simulink model "px4demo_gps"  (R2017b)
settings: Solver=ode3  StartTime=0.0  StopTime=inf  RelTol=1e-3  EnableMultiTasking=on
PostLoadFcn:
  | Ts = 1/250;
undefined symbols (not defined in the file): RGBLED_COLOR_ENUM, RGBLED_MODE_ENUM
libraries: pixhawk_slib_sensors_actuators x2
Description:
  | PX4 PSP Demo Model - GPS
  | 
  | Example model to show how to use the GPS Input Block
settings Model: Creator=skuznick  LastModifiedBy=skuznick
settings SolverCC: PositivePriorityOrder=on
settings DataIOCC: LimitDataPoints=on  SaveFormat=Array
settings OptimizationCC: DefaultParameterBehavior=Inlined  LifeSpan=1  MaxStackSize=64
settings DebuggingCC: SolverPrmCheckMsg=warning  AllowSymbolicDim=off  SFUnexpectedBacktrackingDiag=warning  SFNoUnconditionalDefaultTransitionDiag=warning  SFExecutionAtInitializationDiag=none
settings HardwareCC: ProdBitPerPointer=32  ProdBitPerSizeT=32  ProdBitPerPtrDiffT=32  ProdLargestAtomicInteger=Long  ProdLargestAtomicFloat=Double  ProdWordSize=32  ProdHWDeviceType=ARM Compatible->ARM Cortex
settings ModelReferenceCC: PropagateSignalLabelsOutOfModel=off
settings SFSimCC: MATLABDynamicMemAlloc=off
settings RTWCC: SystemTargetFile=ert.tlc  TemplateMakefile=ert_default_tmf  GenerateReport=on  Toolchain=Pixhawk Toolchain  BuildConfiguration=Faster Runs  IncludeHyperlinkInReport=on  LaunchReport=on  GenerateTraceReport=on  GenerateCodeMetricsReport=on
settings CodeAppCC: IgnoreCustomStorageClasses=off  StateflowObjectComments=on
settings ERTTargetCC: MultiwordLength=2048  ERTCustomFileTemplate=px4_codertarget_file_process.tlc  ConvertIfToSwitch=off  SuppressUnreachableDefaultCases=off
settings ConfigComp: CovMetricSettings=dw  CovHtmlReporting=on  CovSaveCumulativeToWorkspaceVar=on  CovSaveSingleToWorkspaceVar=on  CovExternalEMLEnable=off  CovSFcnEnable=off

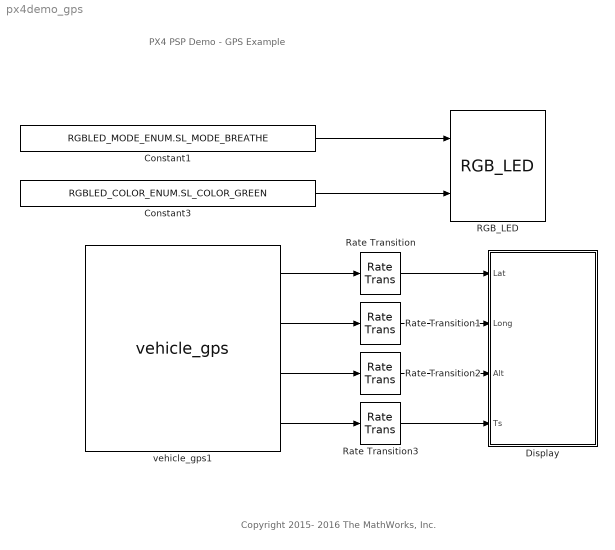
== system px4demo_gps ==
  note: Copyright 2015- 2016 The MathWorks, Inc.
  note: PX4 PSP Demo - GPS Example
  Constant1 : Constant  Value=RGBLED_MODE_ENUM.SL_MODE_BREATHE  OutDataTypeStr=Enum: RGBLED_MODE_ENUM  SampleTime=1
  Constant3 : Constant  Value=RGBLED_COLOR_ENUM.SL_COLOR_GREEN  OutDataTypeStr=Enum: RGBLED_COLOR_ENUM  SampleTime=1
  Display : Subsystem  TreatAsAtomicUnit=on  SystemSampleTime=1
  RGB_LED : pixhawk_slib_sensors_actuators/RGB_LED
      settings: SourceProductName=Pixhawk Target Blocks
  Rate Transition{,1..3} (4 alike) : RateTransition
  vehicle_gps1 : pixhawk_slib_sensors_actuators/vehicle_gps  sampletime=1/250  show_alt=on  show_ts_gps=on  show_vel=off  show_fixtype=off  show_numsat=off
      settings: SourceProductName=Pixhawk Target Blocks
  wires:
  Constant1/1 -> RGB_LED/1
  Constant3/1 -> RGB_LED/2
  vehicle_gps1/1 -> Rate Transition/1
  vehicle_gps1/2 -> Rate Transition1/1
  vehicle_gps1/4 -> Rate Transition3/1
  vehicle_gps1/3 -> Rate Transition2/1
  Rate Transition/1 -> Display/1(Lat)
  Rate Transition1/1 -> Display/2(Long)
  Rate Transition2/1 -> Display/3(Alt)
  Rate Transition3/1 -> Display/4(Ts)

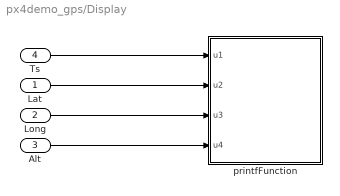
== system px4demo_gps/Display ==
  Lat : Inport
  Long : Inport  Port=2
  Alt : Inport  Port=3
  Ts : Inport  Port=4
  printfFunction : MATLAB Function  TreatAsAtomicUnit=on
  wires:
  Ts/1 -> printfFunction/1(u1)
  Lat/1 -> printfFunction/2(u2)
  Long/1 -> printfFunction/3(u3)
  Alt/1 -> printfFunction/4(u4)

== matlab function px4demo_gps/Display/printfFunction ==
  data: u1 input double; u2 input int32; u3 input int32; u4 input
function fcn(u1, u2, u3,u4)
%#codegen

if strcmp(coder.target, 'rtw') == true
    coder.ceval('printf',['UTC Time GPS->TS: %f ', uint8(10) uint8(0)],   u1);
    coder.ceval('printf',['GPS->LAT: %d ', uint8(10) uint8(0)], int32(u2));
    coder.ceval('printf',['GPS->LON: %d ', uint8(10) uint8(0)], int32(u3));
    coder.ceval('printf',['GPS->ALT: %d ', uint8(10) uint8(0)], int32(u4));

end
